simulink model "gm_soc_dvbs2_fpga"  (R2025b)
settings: Solver=VariableStepAuto  StartTime=0.0  StopTime=10.0  RelTol=1e-3
InitFcn:
  | soc_dvbs2_init;
undefined symbols (not defined in the file or in its folder): Add, coefficientsLog, coefficientsSqrt1, coefficientsSqrt2, dataBits, Deinterleaver, designMultirateFIR, noisePow, Shift, Short, soc_dvbs2_designFIRFilter, soc_dvbs2_txPacketBits, syncWord, txDataOut, txFiltCoeff, XData
libraries: simulink x304, hdlsllib x265, dspsigops x15, dsphdlfiltering2 x8, hdlmdlgenlib x6, dsphdlsigops2 x5, commseqgen3 x5, dsphdlmathfun2 x3, hwlogicconnlib x2, whdledac x2, commhdlcrc x2, whdlutilities x1
(part 31 of 36)

== system gm_soc_dvbs2_fpga/DVBS2/DVBS2 TxRx/DVB-S2 HDL Receiver/Synchronizer and PL Header Decoder/PL Header Recovery/PL Header Decoder/ML Decoder/Get Min Index/For Each Subsystem2_instance6 ==
  note: For Each
  valueIn : Inport  OutDataTypeStr=fixdt(1, 25, 15)  PortDimensions=[2]  SampleTime=2.5e-07
  idxIn : Inport  Port=2  OutDataTypeStr=fixdt(0, 6, 0)  PortDimensions=[2]  SampleTime=2.5e-07
  Delay{1..9} (9 alike) : Delay  DelayLength=double(1)  InitialCondition=0  SampleTime=2.5e-07
  Relational Operator : RelationalOperator  Operator=<  OutDataTypeStr=boolean  SampleTime=2.5e-07  InputSameDT=off
  Switch : Switch  Criteria=u2 ~= 0  Threshold="fi(0,0,1,0,\"hex\",\"0\")"  OutDataTypeStr=fixdt(1, 25, 15)  SampleTime=2.5e-07  SaturateOnIntegerOverflow=off  InputSameDT=off
  Switch1 : Switch  Criteria=u2 ~= 0  Threshold="fi(0,0,1,0,\"hex\",\"0\")"  OutDataTypeStr=fixdt(0, 6, 0)  SampleTime=2.5e-07  SaturateOnIntegerOverflow=off  InputSameDT=off
  t : Demux  Outputs=2
  t1 : Demux  Outputs=2
  ValueOut : Outport  SampleTime=2.5e-07
  idxOut : Outport  Port=2  SampleTime=2.5e-07
  wires:
  valueIn/1 -> Delay3/1
  Delay9/1 -> idxOut/1
  Delay1/1 -> t/1
  Delay3/1 -> t1/1
  idxIn/1 -> Delay1/1
  t1/1 -> Relational Operator/1, Delay4/1
  t1/2 -> Delay5/1, Relational Operator/2
  Relational Operator/1 -> Delay2/1
  Delay4/1 -> Switch/1
  t/1 -> Delay6/1
  t/2 -> Delay7/1
  Delay5/1 -> Switch/3
  Delay2/1 -> Switch/2, Switch1/2
  Delay6/1 -> Switch1/1
  Switch1/1 -> Delay9/1
  Delay7/1 -> Switch1/3
  Delay8/1 -> ValueOut/1
  Switch/1 -> Delay8/1

== system gm_soc_dvbs2_fpga/DVBS2/DVBS2 TxRx/DVB-S2 HDL Receiver/Synchronizer and PL Header Decoder/PL Header Recovery/PL Header Decoder/ML Decoder/Get Min Index/For Each Subsystem2_instance7 ==
  note: For Each
  valueIn : Inport  OutDataTypeStr=fixdt(1, 25, 15)  PortDimensions=[2]  SampleTime=2.5e-07
  idxIn : Inport  Port=2  OutDataTypeStr=fixdt(0, 6, 0)  PortDimensions=[2]  SampleTime=2.5e-07
  Delay{1..9} (9 alike) : Delay  DelayLength=double(1)  InitialCondition=0  SampleTime=2.5e-07
  Relational Operator : RelationalOperator  Operator=<  OutDataTypeStr=boolean  SampleTime=2.5e-07  InputSameDT=off
  Switch : Switch  Criteria=u2 ~= 0  Threshold="fi(0,0,1,0,\"hex\",\"0\")"  OutDataTypeStr=fixdt(1, 25, 15)  SampleTime=2.5e-07  SaturateOnIntegerOverflow=off  InputSameDT=off
  Switch1 : Switch  Criteria=u2 ~= 0  Threshold="fi(0,0,1,0,\"hex\",\"0\")"  OutDataTypeStr=fixdt(0, 6, 0)  SampleTime=2.5e-07  SaturateOnIntegerOverflow=off  InputSameDT=off
  t : Demux  Outputs=2
  t1 : Demux  Outputs=2
  ValueOut : Outport  SampleTime=2.5e-07
  idxOut : Outport  Port=2  SampleTime=2.5e-07
  wires:
  Delay8/1 -> ValueOut/1
  valueIn/1 -> Delay3/1
  idxIn/1 -> Delay1/1
  t/1 -> Delay6/1
  Switch1/1 -> Delay9/1
  t1/1 -> Delay4/1, Relational Operator/1
  Delay1/1 -> t/1
  Delay3/1 -> t1/1
  t/2 -> Delay7/1
  t1/2 -> Relational Operator/2, Delay5/1
  Relational Operator/1 -> Delay2/1
  Delay5/1 -> Switch/3
  Delay6/1 -> Switch1/1
  Delay7/1 -> Switch1/3
  Delay2/1 -> Switch/2, Switch1/2
  Delay4/1 -> Switch/1
  Switch/1 -> Delay8/1
  Delay9/1 -> idxOut/1

== system gm_soc_dvbs2_fpga/DVBS2/DVBS2 TxRx/DVB-S2 HDL Receiver/Synchronizer and PL Header Decoder/PL Header Recovery/PL Header Decoder/ML Decoder/Get Min Index/For Each Subsystem2_instance8 ==
  note: For Each
  valueIn : Inport  OutDataTypeStr=fixdt(1, 25, 15)  PortDimensions=[2]  SampleTime=2.5e-07
  idxIn : Inport  Port=2  OutDataTypeStr=fixdt(0, 6, 0)  PortDimensions=[2]  SampleTime=2.5e-07
  Delay{1..9} (9 alike) : Delay  DelayLength=double(1)  InitialCondition=0  SampleTime=2.5e-07
  Relational Operator : RelationalOperator  Operator=<  OutDataTypeStr=boolean  SampleTime=2.5e-07  InputSameDT=off
  Switch : Switch  Criteria=u2 ~= 0  Threshold="fi(0,0,1,0,\"hex\",\"0\")"  OutDataTypeStr=fixdt(1, 25, 15)  SampleTime=2.5e-07  SaturateOnIntegerOverflow=off  InputSameDT=off
  Switch1 : Switch  Criteria=u2 ~= 0  Threshold="fi(0,0,1,0,\"hex\",\"0\")"  OutDataTypeStr=fixdt(0, 6, 0)  SampleTime=2.5e-07  SaturateOnIntegerOverflow=off  InputSameDT=off
  t : Demux  Outputs=2
  t1 : Demux  Outputs=2
  ValueOut : Outport  SampleTime=2.5e-07
  idxOut : Outport  Port=2  SampleTime=2.5e-07
  wires:
  Delay8/1 -> ValueOut/1
  valueIn/1 -> Delay3/1
  idxIn/1 -> Delay1/1
  t/1 -> Delay6/1
  Switch1/1 -> Delay9/1
  t1/1 -> Delay4/1, Relational Operator/1
  Delay1/1 -> t/1
  Delay3/1 -> t1/1
  t/2 -> Delay7/1
  Delay4/1 -> Switch/1
  t1/2 -> Relational Operator/2, Delay5/1
  Relational Operator/1 -> Delay2/1
  Delay5/1 -> Switch/3
  Delay6/1 -> Switch1/1
  Delay7/1 -> Switch1/3
  Delay2/1 -> Switch/2, Switch1/2
  Switch/1 -> Delay8/1
  Delay9/1 -> idxOut/1

== system gm_soc_dvbs2_fpga/DVBS2/DVBS2 TxRx/DVB-S2 HDL Receiver/Synchronizer and PL Header Decoder/PL Header Recovery/PL Header Decoder/ML Decoder/Get Min Index/For Each Subsystem3_instance1 ==
  note: For Each
  valueIn : Inport  OutDataTypeStr=fixdt(1, 25, 15)  PortDimensions=[2]  SampleTime=2.5e-07
  idxIn : Inport  Port=2  OutDataTypeStr=fixdt(0, 6, 0)  PortDimensions=[2]  SampleTime=2.5e-07
  Delay{1..9} (9 alike) : Delay  DelayLength=double(1)  InitialCondition=0  SampleTime=2.5e-07
  Relational Operator : RelationalOperator  Operator=<  OutDataTypeStr=boolean  SampleTime=2.5e-07  InputSameDT=off
  Switch : Switch  Criteria=u2 ~= 0  Threshold="fi(0,0,1,0,\"hex\",\"0\")"  OutDataTypeStr=fixdt(1, 25, 15)  SampleTime=2.5e-07  SaturateOnIntegerOverflow=off  InputSameDT=off
  Switch1 : Switch  Criteria=u2 ~= 0  Threshold="fi(0,0,1,0,\"hex\",\"0\")"  OutDataTypeStr=fixdt(0, 6, 0)  SampleTime=2.5e-07  SaturateOnIntegerOverflow=off  InputSameDT=off
  t : Demux  Outputs=2
  t1 : Demux  Outputs=2
  ValueOut : Outport  SampleTime=2.5e-07
  idxOut : Outport  Port=2  SampleTime=2.5e-07
  wires:
  Delay4/1 -> Switch/1
  Delay8/1 -> ValueOut/1
  valueIn/1 -> Delay3/1
  Delay1/1 -> t/1
  Delay7/1 -> Switch1/3
  idxIn/1 -> Delay1/1
  Delay3/1 -> t1/1
  Switch1/1 -> Delay9/1
  t1/1 -> Relational Operator/1, Delay4/1
  Relational Operator/1 -> Delay2/1
  t1/2 -> Delay5/1, Relational Operator/2
  t/1 -> Delay6/1
  t/2 -> Delay7/1
  Delay5/1 -> Switch/3
  Delay2/1 -> Switch/2, Switch1/2
  Delay6/1 -> Switch1/1
  Switch/1 -> Delay8/1
  Delay9/1 -> idxOut/1

== system gm_soc_dvbs2_fpga/DVBS2/DVBS2 TxRx/DVB-S2 HDL Receiver/Synchronizer and PL Header Decoder/PL Header Recovery/PL Header Decoder/ML Decoder/Get Min Index/For Each Subsystem3_instance2 ==
  note: For Each
  valueIn : Inport  OutDataTypeStr=fixdt(1, 25, 15)  PortDimensions=[2]  SampleTime=2.5e-07
  idxIn : Inport  Port=2  OutDataTypeStr=fixdt(0, 6, 0)  PortDimensions=[2]  SampleTime=2.5e-07
  Delay{1..9} (9 alike) : Delay  DelayLength=double(1)  InitialCondition=0  SampleTime=2.5e-07
  Relational Operator : RelationalOperator  Operator=<  OutDataTypeStr=boolean  SampleTime=2.5e-07  InputSameDT=off
  Switch : Switch  Criteria=u2 ~= 0  Threshold="fi(0,0,1,0,\"hex\",\"0\")"  OutDataTypeStr=fixdt(1, 25, 15)  SampleTime=2.5e-07  SaturateOnIntegerOverflow=off  InputSameDT=off
  Switch1 : Switch  Criteria=u2 ~= 0  Threshold="fi(0,0,1,0,\"hex\",\"0\")"  OutDataTypeStr=fixdt(0, 6, 0)  SampleTime=2.5e-07  SaturateOnIntegerOverflow=off  InputSameDT=off
  t : Demux  Outputs=2
  t1 : Demux  Outputs=2
  ValueOut : Outport  SampleTime=2.5e-07
  idxOut : Outport  Port=2  SampleTime=2.5e-07
  wires:
  Delay8/1 -> ValueOut/1
  valueIn/1 -> Delay3/1
  Delay1/1 -> t/1
  Switch1/1 -> Delay9/1
  t1/1 -> Relational Operator/1, Delay4/1
  Delay3/1 -> t1/1
  idxIn/1 -> Delay1/1
  Relational Operator/1 -> Delay2/1
  t1/2 -> Delay5/1, Relational Operator/2
  Delay4/1 -> Switch/1
  t/1 -> Delay6/1
  t/2 -> Delay7/1
  Delay5/1 -> Switch/3
  Delay2/1 -> Switch/2, Switch1/2
  Delay6/1 -> Switch1/1
  Delay7/1 -> Switch1/3
  Switch/1 -> Delay8/1
  Delay9/1 -> idxOut/1

== system gm_soc_dvbs2_fpga/DVBS2/DVBS2 TxRx/DVB-S2 HDL Receiver/Synchronizer and PL Header Decoder/PL Header Recovery/PL Header Decoder/ML Decoder/Get Min Index/For Each Subsystem3_instance3 ==
  note: For Each
  valueIn : Inport  OutDataTypeStr=fixdt(1, 25, 15)  PortDimensions=[2]  SampleTime=2.5e-07
  idxIn : Inport  Port=2  OutDataTypeStr=fixdt(0, 6, 0)  PortDimensions=[2]  SampleTime=2.5e-07
  Delay{1..9} (9 alike) : Delay  DelayLength=double(1)  InitialCondition=0  SampleTime=2.5e-07
  Relational Operator : RelationalOperator  Operator=<  OutDataTypeStr=boolean  SampleTime=2.5e-07  InputSameDT=off
  Switch : Switch  Criteria=u2 ~= 0  Threshold="fi(0,0,1,0,\"hex\",\"0\")"  OutDataTypeStr=fixdt(1, 25, 15)  SampleTime=2.5e-07  SaturateOnIntegerOverflow=off  InputSameDT=off
  Switch1 : Switch  Criteria=u2 ~= 0  Threshold="fi(0,0,1,0,\"hex\",\"0\")"  OutDataTypeStr=fixdt(0, 6, 0)  SampleTime=2.5e-07  SaturateOnIntegerOverflow=off  InputSameDT=off
  t : Demux  Outputs=2
  t1 : Demux  Outputs=2
  ValueOut : Outport  SampleTime=2.5e-07
  idxOut : Outport  Port=2  SampleTime=2.5e-07
  wires:
  valueIn/1 -> Delay3/1
  Delay1/1 -> t/1
  Delay3/1 -> t1/1
  idxIn/1 -> Delay1/1
  t1/1 -> Relational Operator/1, Delay4/1
  t1/2 -> Delay5/1, Relational Operator/2
  Relational Operator/1 -> Delay2/1
  Delay4/1 -> Switch/1
  t/1 -> Delay6/1
  t/2 -> Delay7/1
  Delay5/1 -> Switch/3
  Delay2/1 -> Switch/2, Switch1/2
  Delay6/1 -> Switch1/1
  Switch1/1 -> Delay9/1
  Delay7/1 -> Switch1/3
  Delay8/1 -> ValueOut/1
  Switch/1 -> Delay8/1
  Delay9/1 -> idxOut/1

== system gm_soc_dvbs2_fpga/DVBS2/DVBS2 TxRx/DVB-S2 HDL Receiver/Synchronizer and PL Header Decoder/PL Header Recovery/PL Header Decoder/ML Decoder/Get Min Index/For Each Subsystem3_instance4 ==
  note: For Each
  valueIn : Inport  OutDataTypeStr=fixdt(1, 25, 15)  PortDimensions=[2]  SampleTime=2.5e-07
  idxIn : Inport  Port=2  OutDataTypeStr=fixdt(0, 6, 0)  PortDimensions=[2]  SampleTime=2.5e-07
  Delay{1..9} (9 alike) : Delay  DelayLength=double(1)  InitialCondition=0  SampleTime=2.5e-07
  Relational Operator : RelationalOperator  Operator=<  OutDataTypeStr=boolean  SampleTime=2.5e-07  InputSameDT=off
  Switch : Switch  Criteria=u2 ~= 0  Threshold="fi(0,0,1,0,\"hex\",\"0\")"  OutDataTypeStr=fixdt(1, 25, 15)  SampleTime=2.5e-07  SaturateOnIntegerOverflow=off  InputSameDT=off
  Switch1 : Switch  Criteria=u2 ~= 0  Threshold="fi(0,0,1,0,\"hex\",\"0\")"  OutDataTypeStr=fixdt(0, 6, 0)  SampleTime=2.5e-07  SaturateOnIntegerOverflow=off  InputSameDT=off
  t : Demux  Outputs=2
  t1 : Demux  Outputs=2
  ValueOut : Outport  SampleTime=2.5e-07
  idxOut : Outport  Port=2  SampleTime=2.5e-07
  wires:
  Delay8/1 -> ValueOut/1
  valueIn/1 -> Delay3/1
  Delay3/1 -> t1/1
  idxIn/1 -> Delay1/1
  t/1 -> Delay6/1
  Switch1/1 -> Delay9/1
  t1/1 -> Delay4/1, Relational Operator/1
  Delay1/1 -> t/1
  t/2 -> Delay7/1
  t1/2 -> Relational Operator/2, Delay5/1
  Relational Operator/1 -> Delay2/1
  Delay5/1 -> Switch/3
  Delay6/1 -> Switch1/1
  Delay7/1 -> Switch1/3
  Delay2/1 -> Switch/2, Switch1/2
  Delay4/1 -> Switch/1
  Switch/1 -> Delay8/1
  Delay9/1 -> idxOut/1

== system gm_soc_dvbs2_fpga/DVBS2/DVBS2 TxRx/DVB-S2 HDL Receiver/Synchronizer and PL Header Decoder/PL Header Recovery/PL Header Decoder/ML Decoder/Get Min Index/For Each Subsystem4_instance1 ==
  note: For Each
  valueIn : Inport  OutDataTypeStr=fixdt(1, 25, 15)  PortDimensions=[2]  SampleTime=2.5e-07
  idxIn : Inport  Port=2  OutDataTypeStr=fixdt(0, 6, 0)  PortDimensions=[2]  SampleTime=2.5e-07
  Delay{1..9} (9 alike) : Delay  DelayLength=double(1)  InitialCondition=0  SampleTime=2.5e-07
  Relational Operator : RelationalOperator  Operator=<  OutDataTypeStr=boolean  SampleTime=2.5e-07  InputSameDT=off
  Switch : Switch  Criteria=u2 ~= 0  Threshold="fi(0,0,1,0,\"hex\",\"0\")"  OutDataTypeStr=fixdt(1, 25, 15)  SampleTime=2.5e-07  SaturateOnIntegerOverflow=off  InputSameDT=off
  Switch1 : Switch  Criteria=u2 ~= 0  Threshold="fi(0,0,1,0,\"hex\",\"0\")"  OutDataTypeStr=fixdt(0, 6, 0)  SampleTime=2.5e-07  SaturateOnIntegerOverflow=off  InputSameDT=off
  t : Demux  Outputs=2
  t1 : Demux  Outputs=2
  ValueOut : Outport  SampleTime=2.5e-07
  idxOut : Outport  Port=2  SampleTime=2.5e-07
  wires:
  Delay4/1 -> Switch/1
  Delay8/1 -> ValueOut/1
  valueIn/1 -> Delay3/1
  Delay7/1 -> Switch1/3
  idxIn/1 -> Delay1/1
  Delay3/1 -> t1/1
  Delay1/1 -> t/1
  Switch1/1 -> Delay9/1
  t1/1 -> Relational Operator/1, Delay4/1
  Relational Operator/1 -> Delay2/1
  t1/2 -> Delay5/1, Relational Operator/2
  t/1 -> Delay6/1
  t/2 -> Delay7/1
  Delay5/1 -> Switch/3
  Delay2/1 -> Switch/2, Switch1/2
  Delay6/1 -> Switch1/1
  Switch/1 -> Delay8/1
  Delay9/1 -> idxOut/1

== system gm_soc_dvbs2_fpga/DVBS2/DVBS2 TxRx/DVB-S2 HDL Receiver/Synchronizer and PL Header Decoder/PL Header Recovery/PL Header Decoder/ML Decoder/Get Min Index/For Each Subsystem4_instance2 ==
  note: For Each
  valueIn : Inport  OutDataTypeStr=fixdt(1, 25, 15)  PortDimensions=[2]  SampleTime=2.5e-07
  idxIn : Inport  Port=2  OutDataTypeStr=fixdt(0, 6, 0)  PortDimensions=[2]  SampleTime=2.5e-07
  Delay{1..9} (9 alike) : Delay  DelayLength=double(1)  InitialCondition=0  SampleTime=2.5e-07
  Relational Operator : RelationalOperator  Operator=<  OutDataTypeStr=boolean  SampleTime=2.5e-07  InputSameDT=off
  Switch : Switch  Criteria=u2 ~= 0  Threshold="fi(0,0,1,0,\"hex\",\"0\")"  OutDataTypeStr=fixdt(1, 25, 15)  SampleTime=2.5e-07  SaturateOnIntegerOverflow=off  InputSameDT=off
  Switch1 : Switch  Criteria=u2 ~= 0  Threshold="fi(0,0,1,0,\"hex\",\"0\")"  OutDataTypeStr=fixdt(0, 6, 0)  SampleTime=2.5e-07  SaturateOnIntegerOverflow=off  InputSameDT=off
  t : Demux  Outputs=2
  t1 : Demux  Outputs=2
  ValueOut : Outport  SampleTime=2.5e-07
  idxOut : Outport  Port=2  SampleTime=2.5e-07
  wires:
  Delay8/1 -> ValueOut/1
  valueIn/1 -> Delay3/1
  Delay1/1 -> t/1
  Switch1/1 -> Delay9/1
  t1/1 -> Delay4/1, Relational Operator/1
  Delay3/1 -> t1/1
  idxIn/1 -> Delay1/1
  Relational Operator/1 -> Delay2/1
  t1/2 -> Delay5/1, Relational Operator/2
  Delay4/1 -> Switch/1
  t/1 -> Delay6/1
  t/2 -> Delay7/1
  Delay5/1 -> Switch/3
  Delay2/1 -> Switch/2, Switch1/2
  Delay6/1 -> Switch1/1
  Delay7/1 -> Switch1/3
  Switch/1 -> Delay8/1
  Delay9/1 -> idxOut/1

== system gm_soc_dvbs2_fpga/DVBS2/DVBS2 TxRx/DVB-S2 HDL Receiver/Synchronizer and PL Header Decoder/PL Header Recovery/PL Header Decoder/ML Decoder/Get Min Index/For Each Subsystem5 ==
  valueIn : Inport  OutDataTypeStr=fixdt(1, 25, 15)  PortDimensions=[2]  SampleTime=2.5e-07
  idxIn : Inport  Port=2  OutDataTypeStr=fixdt(0, 6, 0)  PortDimensions=[2]  SampleTime=2.5e-07
  Delay{1..6} (6 alike) : Delay  DelayLength=double(1)  InitialCondition=0  SampleTime=2.5e-07
  Relational Operator : RelationalOperator  Operator=<  OutDataTypeStr=boolean  SampleTime=2.5e-07  InputSameDT=off
  Switch1 : Switch  Criteria=u2 ~= 0  Threshold="fi(0,0,1,0,\"hex\",\"0\")"  OutDataTypeStr=fixdt(0, 6, 0)  SampleTime=2.5e-07  SaturateOnIntegerOverflow=off  InputSameDT=off
  t : Demux  Outputs=2
  t1 : Demux  Outputs=2
  idxOut : Outport  SampleTime=2.5e-07
  wires:
  Delay1/1 -> t1/1
  valueIn/1 -> Delay3/1
  Delay3/1 -> t/1
  t1/1 -> Delay2/1
  t/1 -> Relational Operator/1
  idxIn/1 -> Delay1/1
  Relational Operator/1 -> Delay4/1
  t/2 -> Relational Operator/2
  t1/2 -> Delay5/1
  Delay2/1 -> Switch1/1
  Delay4/1 -> Switch1/2
  Delay5/1 -> Switch1/3
  Switch1/1 -> Delay6/1
  Delay6/1 -> idxOut/1

== system gm_soc_dvbs2_fpga/DVBS2/DVBS2 TxRx/DVB-S2 HDL Receiver/Synchronizer and PL Header Decoder/PL Header Recovery/PL Header Decoder/ML Decoder/Get Min Index/For Each Subsystem_instance1 ==
  note: For Each
  valueIn : Inport  OutDataTypeStr=fixdt(1, 25, 15)  PortDimensions=[2]  SampleTime=2.5e-07
  idxIn : Inport  Port=2  OutDataTypeStr=fixdt(0, 6, 0)  PortDimensions=[2]  SampleTime=2.5e-07
  Delay{1..9} (9 alike) : Delay  DelayLength=double(1)  InitialCondition=0  SampleTime=2.5e-07
  Relational Operator : RelationalOperator  Operator=<  OutDataTypeStr=boolean  SampleTime=2.5e-07  InputSameDT=off
  Switch : Switch  Criteria=u2 ~= 0  Threshold="fi(0,0,1,0,\"hex\",\"0\")"  OutDataTypeStr=fixdt(1, 25, 15)  SampleTime=2.5e-07  SaturateOnIntegerOverflow=off  InputSameDT=off
  Switch1 : Switch  Criteria=u2 ~= 0  Threshold="fi(0,0,1,0,\"hex\",\"0\")"  OutDataTypeStr=fixdt(0, 6, 0)  SampleTime=2.5e-07  SaturateOnIntegerOverflow=off  InputSameDT=off
  t : Demux  Outputs=2
  t1 : Demux  Outputs=2
  ValueOut : Outport  SampleTime=2.5e-07
  idxOut : Outport  Port=2  SampleTime=2.5e-07
  wires:
  valueIn/1 -> Delay3/1
  Delay9/1 -> idxOut/1
  Delay1/1 -> t/1
  Switch1/1 -> Delay9/1
  t1/1 -> Relational Operator/1, Delay4/1
  Delay3/1 -> t1/1
  idxIn/1 -> Delay1/1
  Relational Operator/1 -> Delay2/1
  t1/2 -> Delay5/1, Relational Operator/2
  Delay4/1 -> Switch/1
  t/1 -> Delay6/1
  t/2 -> Delay7/1
  Delay5/1 -> Switch/3
  Delay2/1 -> Switch1/2, Switch/2
  Delay6/1 -> Switch1/1
  Delay7/1 -> Switch1/3
  Delay8/1 -> ValueOut/1
  Switch/1 -> Delay8/1

== system gm_soc_dvbs2_fpga/DVBS2/DVBS2 TxRx/DVB-S2 HDL Receiver/Synchronizer and PL Header Decoder/PL Header Recovery/PL Header Decoder/ML Decoder/Get Min Index/For Each Subsystem_instance10 ==
  note: For Each
  valueIn : Inport  OutDataTypeStr=fixdt(1, 25, 15)  PortDimensions=[2]  SampleTime=2.5e-07
  idxIn : Inport  Port=2  OutDataTypeStr=fixdt(0, 6, 0)  PortDimensions=[2]  SampleTime=2.5e-07
  Delay{1..9} (9 alike) : Delay  DelayLength=double(1)  InitialCondition=0  SampleTime=2.5e-07
  Relational Operator : RelationalOperator  Operator=<  OutDataTypeStr=boolean  SampleTime=2.5e-07  InputSameDT=off
  Switch : Switch  Criteria=u2 ~= 0  Threshold="fi(0,0,1,0,\"hex\",\"0\")"  OutDataTypeStr=fixdt(1, 25, 15)  SampleTime=2.5e-07  SaturateOnIntegerOverflow=off  InputSameDT=off
  Switch1 : Switch  Criteria=u2 ~= 0  Threshold="fi(0,0,1,0,\"hex\",\"0\")"  OutDataTypeStr=fixdt(0, 6, 0)  SampleTime=2.5e-07  SaturateOnIntegerOverflow=off  InputSameDT=off
  t : Demux  Outputs=2
  t1 : Demux  Outputs=2
  ValueOut : Outport  SampleTime=2.5e-07
  idxOut : Outport  Port=2  SampleTime=2.5e-07
  wires:
  Delay8/1 -> ValueOut/1
  valueIn/1 -> Delay3/1
  Delay1/1 -> t/1
  Switch1/1 -> Delay9/1
  t1/1 -> Relational Operator/1, Delay4/1
  Delay3/1 -> t1/1
  idxIn/1 -> Delay1/1
  Relational Operator/1 -> Delay2/1
  t1/2 -> Delay5/1, Relational Operator/2
  Delay4/1 -> Switch/1
  t/1 -> Delay6/1
  t/2 -> Delay7/1
  Delay5/1 -> Switch/3
  Delay2/1 -> Switch/2, Switch1/2
  Delay6/1 -> Switch1/1
  Delay7/1 -> Switch1/3
  Switch/1 -> Delay8/1
  Delay9/1 -> idxOut/1

== system gm_soc_dvbs2_fpga/DVBS2/DVBS2 TxRx/DVB-S2 HDL Receiver/Synchronizer and PL Header Decoder/PL Header Recovery/PL Header Decoder/ML Decoder/Get Min Index/For Each Subsystem_instance11 ==
  note: For Each
  valueIn : Inport  OutDataTypeStr=fixdt(1, 25, 15)  PortDimensions=[2]  SampleTime=2.5e-07
  idxIn : Inport  Port=2  OutDataTypeStr=fixdt(0, 6, 0)  PortDimensions=[2]  SampleTime=2.5e-07
  Delay{1..9} (9 alike) : Delay  DelayLength=double(1)  InitialCondition=0  SampleTime=2.5e-07
  Relational Operator : RelationalOperator  Operator=<  OutDataTypeStr=boolean  SampleTime=2.5e-07  InputSameDT=off
  Switch : Switch  Criteria=u2 ~= 0  Threshold="fi(0,0,1,0,\"hex\",\"0\")"  OutDataTypeStr=fixdt(1, 25, 15)  SampleTime=2.5e-07  SaturateOnIntegerOverflow=off  InputSameDT=off
  Switch1 : Switch  Criteria=u2 ~= 0  Threshold="fi(0,0,1,0,\"hex\",\"0\")"  OutDataTypeStr=fixdt(0, 6, 0)  SampleTime=2.5e-07  SaturateOnIntegerOverflow=off  InputSameDT=off
  t : Demux  Outputs=2
  t1 : Demux  Outputs=2
  ValueOut : Outport  SampleTime=2.5e-07
  idxOut : Outport  Port=2  SampleTime=2.5e-07
  wires:
  Delay8/1 -> ValueOut/1
  valueIn/1 -> Delay3/1
  Delay9/1 -> idxOut/1
  Delay1/1 -> t/1
  Delay3/1 -> t1/1
  idxIn/1 -> Delay1/1
  t/1 -> Delay6/1
  Switch1/1 -> Delay9/1
  t1/1 -> Delay4/1, Relational Operator/1
  t/2 -> Delay7/1
  t1/2 -> Relational Operator/2, Delay5/1
  Relational Operator/1 -> Delay2/1
  Delay5/1 -> Switch/3
  Delay6/1 -> Switch1/1
  Delay7/1 -> Switch1/3
  Delay2/1 -> Switch/2, Switch1/2
  Delay4/1 -> Switch/1
  Switch/1 -> Delay8/1

== system gm_soc_dvbs2_fpga/DVBS2/DVBS2 TxRx/DVB-S2 HDL Receiver/Synchronizer and PL Header Decoder/PL Header Recovery/PL Header Decoder/ML Decoder/Get Min Index/For Each Subsystem_instance12 ==
  note: For Each
  valueIn : Inport  OutDataTypeStr=fixdt(1, 25, 15)  PortDimensions=[2]  SampleTime=2.5e-07
  idxIn : Inport  Port=2  OutDataTypeStr=fixdt(0, 6, 0)  PortDimensions=[2]  SampleTime=2.5e-07
  Delay{1..9} (9 alike) : Delay  DelayLength=double(1)  InitialCondition=0  SampleTime=2.5e-07
  Relational Operator : RelationalOperator  Operator=<  OutDataTypeStr=boolean  SampleTime=2.5e-07  InputSameDT=off
  Switch : Switch  Criteria=u2 ~= 0  Threshold="fi(0,0,1,0,\"hex\",\"0\")"  OutDataTypeStr=fixdt(1, 25, 15)  SampleTime=2.5e-07  SaturateOnIntegerOverflow=off  InputSameDT=off
  Switch1 : Switch  Criteria=u2 ~= 0  Threshold="fi(0,0,1,0,\"hex\",\"0\")"  OutDataTypeStr=fixdt(0, 6, 0)  SampleTime=2.5e-07  SaturateOnIntegerOverflow=off  InputSameDT=off
  t : Demux  Outputs=2
  t1 : Demux  Outputs=2
  ValueOut : Outport  SampleTime=2.5e-07
  idxOut : Outport  Port=2  SampleTime=2.5e-07
  wires:
  Delay8/1 -> ValueOut/1
  valueIn/1 -> Delay3/1
  Delay1/1 -> t/1
  Switch1/1 -> Delay9/1
  t1/1 -> Relational Operator/1, Delay4/1
  Delay3/1 -> t1/1
  idxIn/1 -> Delay1/1
  Relational Operator/1 -> Delay2/1
  t1/2 -> Delay5/1, Relational Operator/2
  Delay4/1 -> Switch/1
  t/1 -> Delay6/1
  t/2 -> Delay7/1
  Delay5/1 -> Switch/3
  Delay2/1 -> Switch/2, Switch1/2
  Delay6/1 -> Switch1/1
  Delay7/1 -> Switch1/3
  Switch/1 -> Delay8/1
  Delay9/1 -> idxOut/1

== system gm_soc_dvbs2_fpga/DVBS2/DVBS2 TxRx/DVB-S2 HDL Receiver/Synchronizer and PL Header Decoder/PL Header Recovery/PL Header Decoder/ML Decoder/Get Min Index/For Each Subsystem_instance13 ==
  note: For Each
  valueIn : Inport  OutDataTypeStr=fixdt(1, 25, 15)  PortDimensions=[2]  SampleTime=2.5e-07
  idxIn : Inport  Port=2  OutDataTypeStr=fixdt(0, 6, 0)  PortDimensions=[2]  SampleTime=2.5e-07
  Delay{1..9} (9 alike) : Delay  DelayLength=double(1)  InitialCondition=0  SampleTime=2.5e-07
  Relational Operator : RelationalOperator  Operator=<  OutDataTypeStr=boolean  SampleTime=2.5e-07  InputSameDT=off
  Switch : Switch  Criteria=u2 ~= 0  Threshold="fi(0,0,1,0,\"hex\",\"0\")"  OutDataTypeStr=fixdt(1, 25, 15)  SampleTime=2.5e-07  SaturateOnIntegerOverflow=off  InputSameDT=off
  Switch1 : Switch  Criteria=u2 ~= 0  Threshold="fi(0,0,1,0,\"hex\",\"0\")"  OutDataTypeStr=fixdt(0, 6, 0)  SampleTime=2.5e-07  SaturateOnIntegerOverflow=off  InputSameDT=off
  t : Demux  Outputs=2
  t1 : Demux  Outputs=2
  ValueOut : Outport  SampleTime=2.5e-07
  idxOut : Outport  Port=2  SampleTime=2.5e-07
  wires:
  valueIn/1 -> Delay3/1
  idxIn/1 -> Delay1/1
  t/1 -> Delay6/1
  Delay1/1 -> t/1
  Delay3/1 -> t1/1
  t1/1 -> Delay4/1, Relational Operator/1
  t/2 -> Delay7/1
  t1/2 -> Relational Operator/2, Delay5/1
  Relational Operator/1 -> Delay2/1
  Delay5/1 -> Switch/3
  Delay6/1 -> Switch1/1
  Switch1/1 -> Delay9/1
  Delay7/1 -> Switch1/3
  Delay2/1 -> Switch/2, Switch1/2
  Delay4/1 -> Switch/1
  Delay8/1 -> ValueOut/1
  Switch/1 -> Delay8/1
  Delay9/1 -> idxOut/1

== system gm_soc_dvbs2_fpga/DVBS2/DVBS2 TxRx/DVB-S2 HDL Receiver/Synchronizer and PL Header Decoder/PL Header Recovery/PL Header Decoder/ML Decoder/Get Min Index/For Each Subsystem_instance14 ==
  note: For Each
  valueIn : Inport  OutDataTypeStr=fixdt(1, 25, 15)  PortDimensions=[2]  SampleTime=2.5e-07
  idxIn : Inport  Port=2  OutDataTypeStr=fixdt(0, 6, 0)  PortDimensions=[2]  SampleTime=2.5e-07
  Delay{1..9} (9 alike) : Delay  DelayLength=double(1)  InitialCondition=0  SampleTime=2.5e-07
  Relational Operator : RelationalOperator  Operator=<  OutDataTypeStr=boolean  SampleTime=2.5e-07  InputSameDT=off
  Switch : Switch  Criteria=u2 ~= 0  Threshold="fi(0,0,1,0,\"hex\",\"0\")"  OutDataTypeStr=fixdt(1, 25, 15)  SampleTime=2.5e-07  SaturateOnIntegerOverflow=off  InputSameDT=off
  Switch1 : Switch  Criteria=u2 ~= 0  Threshold="fi(0,0,1,0,\"hex\",\"0\")"  OutDataTypeStr=fixdt(0, 6, 0)  SampleTime=2.5e-07  SaturateOnIntegerOverflow=off  InputSameDT=off
  t : Demux  Outputs=2
  t1 : Demux  Outputs=2
  ValueOut : Outport  SampleTime=2.5e-07
  idxOut : Outport  Port=2  SampleTime=2.5e-07
  wires:
  Delay8/1 -> ValueOut/1
  valueIn/1 -> Delay3/1
  Delay3/1 -> t1/1
  idxIn/1 -> Delay1/1
  t/1 -> Delay6/1
  Switch1/1 -> Delay9/1
  t1/1 -> Delay4/1, Relational Operator/1
  Delay1/1 -> t/1
  t/2 -> Delay7/1
  t1/2 -> Relational Operator/2, Delay5/1
  Relational Operator/1 -> Delay2/1
  Delay5/1 -> Switch/3
  Delay6/1 -> Switch1/1
  Delay7/1 -> Switch1/3
  Delay2/1 -> Switch/2, Switch1/2
  Delay4/1 -> Switch/1
  Switch/1 -> Delay8/1
  Delay9/1 -> idxOut/1

== system gm_soc_dvbs2_fpga/DVBS2/DVBS2 TxRx/DVB-S2 HDL Receiver/Synchronizer and PL Header Decoder/PL Header Recovery/PL Header Decoder/ML Decoder/Get Min Index/For Each Subsystem_instance15 ==
  note: For Each
  valueIn : Inport  OutDataTypeStr=fixdt(1, 25, 15)  PortDimensions=[2]  SampleTime=2.5e-07
  idxIn : Inport  Port=2  OutDataTypeStr=fixdt(0, 6, 0)  PortDimensions=[2]  SampleTime=2.5e-07
  Delay{1..9} (9 alike) : Delay  DelayLength=double(1)  InitialCondition=0  SampleTime=2.5e-07
  Relational Operator : RelationalOperator  Operator=<  OutDataTypeStr=boolean  SampleTime=2.5e-07  InputSameDT=off
  Switch : Switch  Criteria=u2 ~= 0  Threshold="fi(0,0,1,0,\"hex\",\"0\")"  OutDataTypeStr=fixdt(1, 25, 15)  SampleTime=2.5e-07  SaturateOnIntegerOverflow=off  InputSameDT=off
  Switch1 : Switch  Criteria=u2 ~= 0  Threshold="fi(0,0,1,0,\"hex\",\"0\")"  OutDataTypeStr=fixdt(0, 6, 0)  SampleTime=2.5e-07  SaturateOnIntegerOverflow=off  InputSameDT=off
  t : Demux  Outputs=2
  t1 : Demux  Outputs=2
  ValueOut : Outport  SampleTime=2.5e-07
  idxOut : Outport  Port=2  SampleTime=2.5e-07
  wires:
  Delay8/1 -> ValueOut/1
  valueIn/1 -> Delay3/1
  Delay1/1 -> t/1
  Switch1/1 -> Delay9/1
  t1/1 -> Relational Operator/1, Delay4/1
  Delay3/1 -> t1/1
  idxIn/1 -> Delay1/1
  Relational Operator/1 -> Delay2/1
  t1/2 -> Delay5/1, Relational Operator/2
  Delay4/1 -> Switch/1
  t/1 -> Delay6/1
  t/2 -> Delay7/1
  Delay5/1 -> Switch/3
  Delay2/1 -> Switch1/2, Switch/2
  Delay6/1 -> Switch1/1
  Delay7/1 -> Switch1/3
  Switch/1 -> Delay8/1
  Delay9/1 -> idxOut/1

== system gm_soc_dvbs2_fpga/DVBS2/DVBS2 TxRx/DVB-S2 HDL Receiver/Synchronizer and PL Header Decoder/PL Header Recovery/PL Header Decoder/ML Decoder/Get Min Index/For Each Subsystem_instance16 ==
  note: For Each
  valueIn : Inport  OutDataTypeStr=fixdt(1, 25, 15)  PortDimensions=[2]  SampleTime=2.5e-07
  idxIn : Inport  Port=2  OutDataTypeStr=fixdt(0, 6, 0)  PortDimensions=[2]  SampleTime=2.5e-07
  Delay{1..9} (9 alike) : Delay  DelayLength=double(1)  InitialCondition=0  SampleTime=2.5e-07
  Relational Operator : RelationalOperator  Operator=<  OutDataTypeStr=boolean  SampleTime=2.5e-07  InputSameDT=off
  Switch : Switch  Criteria=u2 ~= 0  Threshold="fi(0,0,1,0,\"hex\",\"0\")"  OutDataTypeStr=fixdt(1, 25, 15)  SampleTime=2.5e-07  SaturateOnIntegerOverflow=off  InputSameDT=off
  Switch1 : Switch  Criteria=u2 ~= 0  Threshold="fi(0,0,1,0,\"hex\",\"0\")"  OutDataTypeStr=fixdt(0, 6, 0)  SampleTime=2.5e-07  SaturateOnIntegerOverflow=off  InputSameDT=off
  t : Demux  Outputs=2
  t1 : Demux  Outputs=2
  ValueOut : Outport  SampleTime=2.5e-07
  idxOut : Outport  Port=2  SampleTime=2.5e-07
  wires:
  valueIn/1 -> Delay3/1
  Delay9/1 -> idxOut/1
  Delay1/1 -> t/1
  Delay3/1 -> t1/1
  idxIn/1 -> Delay1/1
  t1/1 -> Relational Operator/1, Delay4/1
  Relational Operator/1 -> Delay2/1
  t1/2 -> Delay5/1, Relational Operator/2
  Delay4/1 -> Switch/1
  t/1 -> Delay6/1
  t/2 -> Delay7/1
  Delay5/1 -> Switch/3
  Delay2/1 -> Switch/2, Switch1/2
  Delay6/1 -> Switch1/1
  Switch1/1 -> Delay9/1
  Delay7/1 -> Switch1/3
  Delay8/1 -> ValueOut/1
  Switch/1 -> Delay8/1

== system gm_soc_dvbs2_fpga/DVBS2/DVBS2 TxRx/DVB-S2 HDL Receiver/Synchronizer and PL Header Decoder/PL Header Recovery/PL Header Decoder/ML Decoder/Get Min Index/For Each Subsystem_instance17 ==
  note: For Each
  valueIn : Inport  OutDataTypeStr=fixdt(1, 25, 15)  PortDimensions=[2]  SampleTime=2.5e-07
  idxIn : Inport  Port=2  OutDataTypeStr=fixdt(0, 6, 0)  PortDimensions=[2]  SampleTime=2.5e-07
  Delay{1..9} (9 alike) : Delay  DelayLength=double(1)  InitialCondition=0  SampleTime=2.5e-07
  Relational Operator : RelationalOperator  Operator=<  OutDataTypeStr=boolean  SampleTime=2.5e-07  InputSameDT=off
  Switch : Switch  Criteria=u2 ~= 0  Threshold="fi(0,0,1,0,\"hex\",\"0\")"  OutDataTypeStr=fixdt(1, 25, 15)  SampleTime=2.5e-07  SaturateOnIntegerOverflow=off  InputSameDT=off
  Switch1 : Switch  Criteria=u2 ~= 0  Threshold="fi(0,0,1,0,\"hex\",\"0\")"  OutDataTypeStr=fixdt(0, 6, 0)  SampleTime=2.5e-07  SaturateOnIntegerOverflow=off  InputSameDT=off
  t : Demux  Outputs=2
  t1 : Demux  Outputs=2
  ValueOut : Outport  SampleTime=2.5e-07
  idxOut : Outport  Port=2  SampleTime=2.5e-07
  wires:
  Delay8/1 -> ValueOut/1
  valueIn/1 -> Delay3/1
  Delay1/1 -> t/1
  Switch1/1 -> Delay9/1
  t1/1 -> Relational Operator/1, Delay4/1
  Delay3/1 -> t1/1
  idxIn/1 -> Delay1/1
  Relational Operator/1 -> Delay2/1
  t1/2 -> Delay5/1, Relational Operator/2
  Delay4/1 -> Switch/1
  t/1 -> Delay6/1
  t/2 -> Delay7/1
  Delay5/1 -> Switch/3
  Delay2/1 -> Switch/2, Switch1/2
  Delay6/1 -> Switch1/1
  Delay7/1 -> Switch1/3
  Switch/1 -> Delay8/1
  Delay9/1 -> idxOut/1

== system gm_soc_dvbs2_fpga/DVBS2/DVBS2 TxRx/DVB-S2 HDL Receiver/Synchronizer and PL Header Decoder/PL Header Recovery/PL Header Decoder/ML Decoder/Get Min Index/For Each Subsystem_instance18 ==
  note: For Each
  valueIn : Inport  OutDataTypeStr=fixdt(1, 25, 15)  PortDimensions=[2]  SampleTime=2.5e-07
  idxIn : Inport  Port=2  OutDataTypeStr=fixdt(0, 6, 0)  PortDimensions=[2]  SampleTime=2.5e-07
  Delay{1..9} (9 alike) : Delay  DelayLength=double(1)  InitialCondition=0  SampleTime=2.5e-07
  Relational Operator : RelationalOperator  Operator=<  OutDataTypeStr=boolean  SampleTime=2.5e-07  InputSameDT=off
  Switch : Switch  Criteria=u2 ~= 0  Threshold="fi(0,0,1,0,\"hex\",\"0\")"  OutDataTypeStr=fixdt(1, 25, 15)  SampleTime=2.5e-07  SaturateOnIntegerOverflow=off  InputSameDT=off
  Switch1 : Switch  Criteria=u2 ~= 0  Threshold="fi(0,0,1,0,\"hex\",\"0\")"  OutDataTypeStr=fixdt(0, 6, 0)  SampleTime=2.5e-07  SaturateOnIntegerOverflow=off  InputSameDT=off
  t : Demux  Outputs=2
  t1 : Demux  Outputs=2
  ValueOut : Outport  SampleTime=2.5e-07
  idxOut : Outport  Port=2  SampleTime=2.5e-07
  wires:
  Delay8/1 -> ValueOut/1
  valueIn/1 -> Delay3/1
  Delay1/1 -> t/1
  Switch1/1 -> Delay9/1
  t1/1 -> Relational Operator/1, Delay4/1
  Delay3/1 -> t1/1
  idxIn/1 -> Delay1/1
  Relational Operator/1 -> Delay2/1
  t1/2 -> Delay5/1, Relational Operator/2
  Delay4/1 -> Switch/1
  t/1 -> Delay6/1
  t/2 -> Delay7/1
  Delay5/1 -> Switch/3
  Delay2/1 -> Switch/2, Switch1/2
  Delay6/1 -> Switch1/1
  Delay7/1 -> Switch1/3
  Switch/1 -> Delay8/1
  Delay9/1 -> idxOut/1

== system gm_soc_dvbs2_fpga/DVBS2/DVBS2 TxRx/DVB-S2 HDL Receiver/Synchronizer and PL Header Decoder/PL Header Recovery/PL Header Decoder/ML Decoder/Get Min Index/For Each Subsystem_instance19 ==
  note: For Each
  valueIn : Inport  OutDataTypeStr=fixdt(1, 25, 15)  PortDimensions=[2]  SampleTime=2.5e-07
  idxIn : Inport  Port=2  OutDataTypeStr=fixdt(0, 6, 0)  PortDimensions=[2]  SampleTime=2.5e-07
  Delay{1..9} (9 alike) : Delay  DelayLength=double(1)  InitialCondition=0  SampleTime=2.5e-07
  Relational Operator : RelationalOperator  Operator=<  OutDataTypeStr=boolean  SampleTime=2.5e-07  InputSameDT=off
  Switch : Switch  Criteria=u2 ~= 0  Threshold="fi(0,0,1,0,\"hex\",\"0\")"  OutDataTypeStr=fixdt(1, 25, 15)  SampleTime=2.5e-07  SaturateOnIntegerOverflow=off  InputSameDT=off
  Switch1 : Switch  Criteria=u2 ~= 0  Threshold="fi(0,0,1,0,\"hex\",\"0\")"  OutDataTypeStr=fixdt(0, 6, 0)  SampleTime=2.5e-07  SaturateOnIntegerOverflow=off  InputSameDT=off
  t : Demux  Outputs=2
  t1 : Demux  Outputs=2
  ValueOut : Outport  SampleTime=2.5e-07
  idxOut : Outport  Port=2  SampleTime=2.5e-07
  wires:
  valueIn/1 -> Delay3/1
  idxIn/1 -> Delay1/1
  Delay9/1 -> idxOut/1
  Delay1/1 -> t/1
  Delay3/1 -> t1/1
  t/1 -> Delay6/1
  t1/1 -> Delay4/1, Relational Operator/1
  t/2 -> Delay7/1
  t1/2 -> Relational Operator/2, Delay5/1
  Relational Operator/1 -> Delay2/1
  Delay5/1 -> Switch/3
  Delay6/1 -> Switch1/1
  Switch1/1 -> Delay9/1
  Delay7/1 -> Switch1/3
  Delay2/1 -> Switch/2, Switch1/2
  Delay4/1 -> Switch/1
  Switch/1 -> Delay8/1
  Delay8/1 -> ValueOut/1

== system gm_soc_dvbs2_fpga/DVBS2/DVBS2 TxRx/DVB-S2 HDL Receiver/Synchronizer and PL Header Decoder/PL Header Recovery/PL Header Decoder/ML Decoder/Get Min Index/For Each Subsystem_instance2 ==
  note: For Each
  valueIn : Inport  OutDataTypeStr=fixdt(1, 25, 15)  PortDimensions=[2]  SampleTime=2.5e-07
  idxIn : Inport  Port=2  OutDataTypeStr=fixdt(0, 6, 0)  PortDimensions=[2]  SampleTime=2.5e-07
  Delay{1..9} (9 alike) : Delay  DelayLength=double(1)  InitialCondition=0  SampleTime=2.5e-07
  Relational Operator : RelationalOperator  Operator=<  OutDataTypeStr=boolean  SampleTime=2.5e-07  InputSameDT=off
  Switch : Switch  Criteria=u2 ~= 0  Threshold="fi(0,0,1,0,\"hex\",\"0\")"  OutDataTypeStr=fixdt(1, 25, 15)  SampleTime=2.5e-07  SaturateOnIntegerOverflow=off  InputSameDT=off
  Switch1 : Switch  Criteria=u2 ~= 0  Threshold="fi(0,0,1,0,\"hex\",\"0\")"  OutDataTypeStr=fixdt(0, 6, 0)  SampleTime=2.5e-07  SaturateOnIntegerOverflow=off  InputSameDT=off
  t : Demux  Outputs=2
  t1 : Demux  Outputs=2
  ValueOut : Outport  SampleTime=2.5e-07
  idxOut : Outport  Port=2  SampleTime=2.5e-07
  wires:
  valueIn/1 -> Delay3/1
  Delay9/1 -> idxOut/1
  Delay1/1 -> t/1
  Delay3/1 -> t1/1
  idxIn/1 -> Delay1/1
  t1/1 -> Relational Operator/1, Delay4/1
  t1/2 -> Delay5/1, Relational Operator/2
  Relational Operator/1 -> Delay2/1
  Delay4/1 -> Switch/1
  t/1 -> Delay6/1
  t/2 -> Delay7/1
  Delay5/1 -> Switch/3
  Delay2/1 -> Switch/2, Switch1/2
  Delay6/1 -> Switch1/1
  Switch1/1 -> Delay9/1
  Delay7/1 -> Switch1/3
  Delay8/1 -> ValueOut/1
  Switch/1 -> Delay8/1

== system gm_soc_dvbs2_fpga/DVBS2/DVBS2 TxRx/DVB-S2 HDL Receiver/Synchronizer and PL Header Decoder/PL Header Recovery/PL Header Decoder/ML Decoder/Get Min Index/For Each Subsystem_instance20 ==
  note: For Each
  valueIn : Inport  OutDataTypeStr=fixdt(1, 25, 15)  PortDimensions=[2]  SampleTime=2.5e-07
  idxIn : Inport  Port=2  OutDataTypeStr=fixdt(0, 6, 0)  PortDimensions=[2]  SampleTime=2.5e-07
  Delay{1..9} (9 alike) : Delay  DelayLength=double(1)  InitialCondition=0  SampleTime=2.5e-07
  Relational Operator : RelationalOperator  Operator=<  OutDataTypeStr=boolean  SampleTime=2.5e-07  InputSameDT=off
  Switch : Switch  Criteria=u2 ~= 0  Threshold="fi(0,0,1,0,\"hex\",\"0\")"  OutDataTypeStr=fixdt(1, 25, 15)  SampleTime=2.5e-07  SaturateOnIntegerOverflow=off  InputSameDT=off
  Switch1 : Switch  Criteria=u2 ~= 0  Threshold="fi(0,0,1,0,\"hex\",\"0\")"  OutDataTypeStr=fixdt(0, 6, 0)  SampleTime=2.5e-07  SaturateOnIntegerOverflow=off  InputSameDT=off
  t : Demux  Outputs=2
  t1 : Demux  Outputs=2
  ValueOut : Outport  SampleTime=2.5e-07
  idxOut : Outport  Port=2  SampleTime=2.5e-07
  wires:
  Delay8/1 -> ValueOut/1
  valueIn/1 -> Delay3/1
  Delay1/1 -> t/1
  Switch1/1 -> Delay9/1
  t1/1 -> Relational Operator/1, Delay4/1
  Delay3/1 -> t1/1
  idxIn/1 -> Delay1/1
  Relational Operator/1 -> Delay2/1
  t1/2 -> Delay5/1, Relational Operator/2
  Delay4/1 -> Switch/1
  t/1 -> Delay6/1
  t/2 -> Delay7/1
  Delay5/1 -> Switch/3
  Delay2/1 -> Switch/2, Switch1/2
  Delay6/1 -> Switch1/1
  Delay7/1 -> Switch1/3
  Switch/1 -> Delay8/1
  Delay9/1 -> idxOut/1

== system gm_soc_dvbs2_fpga/DVBS2/DVBS2 TxRx/DVB-S2 HDL Receiver/Synchronizer and PL Header Decoder/PL Header Recovery/PL Header Decoder/ML Decoder/Get Min Index/For Each Subsystem_instance21 ==
  note: For Each
  valueIn : Inport  OutDataTypeStr=fixdt(1, 25, 15)  PortDimensions=[2]  SampleTime=2.5e-07
  idxIn : Inport  Port=2  OutDataTypeStr=fixdt(0, 6, 0)  PortDimensions=[2]  SampleTime=2.5e-07
  Delay{1..9} (9 alike) : Delay  DelayLength=double(1)  InitialCondition=0  SampleTime=2.5e-07
  Relational Operator : RelationalOperator  Operator=<  OutDataTypeStr=boolean  SampleTime=2.5e-07  InputSameDT=off
  Switch : Switch  Criteria=u2 ~= 0  Threshold="fi(0,0,1,0,\"hex\",\"0\")"  OutDataTypeStr=fixdt(1, 25, 15)  SampleTime=2.5e-07  SaturateOnIntegerOverflow=off  InputSameDT=off
  Switch1 : Switch  Criteria=u2 ~= 0  Threshold="fi(0,0,1,0,\"hex\",\"0\")"  OutDataTypeStr=fixdt(0, 6, 0)  SampleTime=2.5e-07  SaturateOnIntegerOverflow=off  InputSameDT=off
  t : Demux  Outputs=2
  t1 : Demux  Outputs=2
  ValueOut : Outport  SampleTime=2.5e-07
  idxOut : Outport  Port=2  SampleTime=2.5e-07
  wires:
  Delay8/1 -> ValueOut/1
  valueIn/1 -> Delay3/1
  idxIn/1 -> Delay1/1
  t/1 -> Delay6/1
  Switch1/1 -> Delay9/1
  t1/1 -> Delay4/1, Relational Operator/1
  Delay1/1 -> t/1
  Delay3/1 -> t1/1
  t/2 -> Delay7/1
  Delay4/1 -> Switch/1
  t1/2 -> Relational Operator/2, Delay5/1
  Relational Operator/1 -> Delay2/1
  Delay5/1 -> Switch/3
  Delay6/1 -> Switch1/1
  Delay7/1 -> Switch1/3
  Delay2/1 -> Switch/2, Switch1/2
  Switch/1 -> Delay8/1
  Delay9/1 -> idxOut/1

== system gm_soc_dvbs2_fpga/DVBS2/DVBS2 TxRx/DVB-S2 HDL Receiver/Synchronizer and PL Header Decoder/PL Header Recovery/PL Header Decoder/ML Decoder/Get Min Index/For Each Subsystem_instance22 ==
  note: For Each
  valueIn : Inport  OutDataTypeStr=fixdt(1, 25, 15)  PortDimensions=[2]  SampleTime=2.5e-07
  idxIn : Inport  Port=2  OutDataTypeStr=fixdt(0, 6, 0)  PortDimensions=[2]  SampleTime=2.5e-07
  Delay{1..9} (9 alike) : Delay  DelayLength=double(1)  InitialCondition=0  SampleTime=2.5e-07
  Relational Operator : RelationalOperator  Operator=<  OutDataTypeStr=boolean  SampleTime=2.5e-07  InputSameDT=off
  Switch : Switch  Criteria=u2 ~= 0  Threshold="fi(0,0,1,0,\"hex\",\"0\")"  OutDataTypeStr=fixdt(1, 25, 15)  SampleTime=2.5e-07  SaturateOnIntegerOverflow=off  InputSameDT=off
  Switch1 : Switch  Criteria=u2 ~= 0  Threshold="fi(0,0,1,0,\"hex\",\"0\")"  OutDataTypeStr=fixdt(0, 6, 0)  SampleTime=2.5e-07  SaturateOnIntegerOverflow=off  InputSameDT=off
  t : Demux  Outputs=2
  t1 : Demux  Outputs=2
  ValueOut : Outport  SampleTime=2.5e-07
  idxOut : Outport  Port=2  SampleTime=2.5e-07
  wires:
  valueIn/1 -> Delay3/1
  Delay9/1 -> idxOut/1
  Delay1/1 -> t/1
  idxIn/1 -> Delay1/1
  Delay3/1 -> t1/1
  Switch1/1 -> Delay9/1
  t1/1 -> Relational Operator/1, Delay4/1
  Relational Operator/1 -> Delay2/1
  t1/2 -> Delay5/1, Relational Operator/2
  Delay4/1 -> Switch/1
  t/1 -> Delay6/1
  t/2 -> Delay7/1
  Delay5/1 -> Switch/3
  Delay2/1 -> Switch/2, Switch1/2
  Delay6/1 -> Switch1/1
  Delay7/1 -> Switch1/3
  Switch/1 -> Delay8/1
  Delay8/1 -> ValueOut/1

== system gm_soc_dvbs2_fpga/DVBS2/DVBS2 TxRx/DVB-S2 HDL Receiver/Synchronizer and PL Header Decoder/PL Header Recovery/PL Header Decoder/ML Decoder/Get Min Index/For Each Subsystem_instance23 ==
  note: For Each
  valueIn : Inport  OutDataTypeStr=fixdt(1, 25, 15)  PortDimensions=[2]  SampleTime=2.5e-07
  idxIn : Inport  Port=2  OutDataTypeStr=fixdt(0, 6, 0)  PortDimensions=[2]  SampleTime=2.5e-07
  Delay{1..9} (9 alike) : Delay  DelayLength=double(1)  InitialCondition=0  SampleTime=2.5e-07
  Relational Operator : RelationalOperator  Operator=<  OutDataTypeStr=boolean  SampleTime=2.5e-07  InputSameDT=off
  Switch : Switch  Criteria=u2 ~= 0  Threshold="fi(0,0,1,0,\"hex\",\"0\")"  OutDataTypeStr=fixdt(1, 25, 15)  SampleTime=2.5e-07  SaturateOnIntegerOverflow=off  InputSameDT=off
  Switch1 : Switch  Criteria=u2 ~= 0  Threshold="fi(0,0,1,0,\"hex\",\"0\")"  OutDataTypeStr=fixdt(0, 6, 0)  SampleTime=2.5e-07  SaturateOnIntegerOverflow=off  InputSameDT=off
  t : Demux  Outputs=2
  t1 : Demux  Outputs=2
  ValueOut : Outport  SampleTime=2.5e-07
  idxOut : Outport  Port=2  SampleTime=2.5e-07
  wires:
  Delay8/1 -> ValueOut/1
  valueIn/1 -> Delay3/1
  idxIn/1 -> Delay1/1
  t/1 -> Delay6/1
  Switch1/1 -> Delay9/1
  t1/1 -> Delay4/1, Relational Operator/1
  Delay1/1 -> t/1
  Delay3/1 -> t1/1
  t/2 -> Delay7/1
  Delay4/1 -> Switch/1
  t1/2 -> Relational Operator/2, Delay5/1
  Relational Operator/1 -> Delay2/1
  Delay5/1 -> Switch/3
  Delay6/1 -> Switch1/1
  Delay7/1 -> Switch1/3
  Delay2/1 -> Switch/2, Switch1/2
  Switch/1 -> Delay8/1
  Delay9/1 -> idxOut/1

== system gm_soc_dvbs2_fpga/DVBS2/DVBS2 TxRx/DVB-S2 HDL Receiver/Synchronizer and PL Header Decoder/PL Header Recovery/PL Header Decoder/ML Decoder/Get Min Index/For Each Subsystem_instance24 ==
  note: For Each
  valueIn : Inport  OutDataTypeStr=fixdt(1, 25, 15)  PortDimensions=[2]  SampleTime=2.5e-07
  idxIn : Inport  Port=2  OutDataTypeStr=fixdt(0, 6, 0)  PortDimensions=[2]  SampleTime=2.5e-07
  Delay{1..9} (9 alike) : Delay  DelayLength=double(1)  InitialCondition=0  SampleTime=2.5e-07
  Relational Operator : RelationalOperator  Operator=<  OutDataTypeStr=boolean  SampleTime=2.5e-07  InputSameDT=off
  Switch : Switch  Criteria=u2 ~= 0  Threshold="fi(0,0,1,0,\"hex\",\"0\")"  OutDataTypeStr=fixdt(1, 25, 15)  SampleTime=2.5e-07  SaturateOnIntegerOverflow=off  InputSameDT=off
  Switch1 : Switch  Criteria=u2 ~= 0  Threshold="fi(0,0,1,0,\"hex\",\"0\")"  OutDataTypeStr=fixdt(0, 6, 0)  SampleTime=2.5e-07  SaturateOnIntegerOverflow=off  InputSameDT=off
  t : Demux  Outputs=2
  t1 : Demux  Outputs=2
  ValueOut : Outport  SampleTime=2.5e-07
  idxOut : Outport  Port=2  SampleTime=2.5e-07
  wires:
  Delay8/1 -> ValueOut/1
  valueIn/1 -> Delay3/1
  Delay1/1 -> t/1
  Delay3/1 -> t1/1
  idxIn/1 -> Delay1/1
  t1/1 -> Relational Operator/1, Delay4/1
  t1/2 -> Delay5/1, Relational Operator/2
  Relational Operator/1 -> Delay2/1
  Delay4/1 -> Switch/1
  t/1 -> Delay6/1
  t/2 -> Delay7/1
  Delay5/1 -> Switch/3
  Delay2/1 -> Switch1/2, Switch/2
  Delay6/1 -> Switch1/1
  Switch1/1 -> Delay9/1
  Delay7/1 -> Switch1/3
  Switch/1 -> Delay8/1
  Delay9/1 -> idxOut/1

== system gm_soc_dvbs2_fpga/DVBS2/DVBS2 TxRx/DVB-S2 HDL Receiver/Synchronizer and PL Header Decoder/PL Header Recovery/PL Header Decoder/ML Decoder/Get Min Index/For Each Subsystem_instance25 ==
  note: For Each
  valueIn : Inport  OutDataTypeStr=fixdt(1, 25, 15)  PortDimensions=[2]  SampleTime=2.5e-07
  idxIn : Inport  Port=2  OutDataTypeStr=fixdt(0, 6, 0)  PortDimensions=[2]  SampleTime=2.5e-07
  Delay{1..9} (9 alike) : Delay  DelayLength=double(1)  InitialCondition=0  SampleTime=2.5e-07
  Relational Operator : RelationalOperator  Operator=<  OutDataTypeStr=boolean  SampleTime=2.5e-07  InputSameDT=off
  Switch : Switch  Criteria=u2 ~= 0  Threshold="fi(0,0,1,0,\"hex\",\"0\")"  OutDataTypeStr=fixdt(1, 25, 15)  SampleTime=2.5e-07  SaturateOnIntegerOverflow=off  InputSameDT=off
  Switch1 : Switch  Criteria=u2 ~= 0  Threshold="fi(0,0,1,0,\"hex\",\"0\")"  OutDataTypeStr=fixdt(0, 6, 0)  SampleTime=2.5e-07  SaturateOnIntegerOverflow=off  InputSameDT=off
  t : Demux  Outputs=2
  t1 : Demux  Outputs=2
  ValueOut : Outport  SampleTime=2.5e-07
  idxOut : Outport  Port=2  SampleTime=2.5e-07
  wires:
  Delay4/1 -> Switch/1
  Delay8/1 -> ValueOut/1
  valueIn/1 -> Delay3/1
  idxIn/1 -> Delay1/1
  Delay3/1 -> t1/1
  Delay1/1 -> t/1
  Switch1/1 -> Delay9/1
  t1/1 -> Delay4/1, Relational Operator/1
  Relational Operator/1 -> Delay2/1
  t1/2 -> Delay5/1, Relational Operator/2
  t/1 -> Delay6/1
  t/2 -> Delay7/1
  Delay5/1 -> Switch/3
  Delay2/1 -> Switch/2, Switch1/2
  Delay6/1 -> Switch1/1
  Delay7/1 -> Switch1/3
  Switch/1 -> Delay8/1
  Delay9/1 -> idxOut/1

== system gm_soc_dvbs2_fpga/DVBS2/DVBS2 TxRx/DVB-S2 HDL Receiver/Synchronizer and PL Header Decoder/PL Header Recovery/PL Header Decoder/ML Decoder/Get Min Index/For Each Subsystem_instance26 ==
  note: For Each
  valueIn : Inport  OutDataTypeStr=fixdt(1, 25, 15)  PortDimensions=[2]  SampleTime=2.5e-07
  idxIn : Inport  Port=2  OutDataTypeStr=fixdt(0, 6, 0)  PortDimensions=[2]  SampleTime=2.5e-07
  Delay{1..9} (9 alike) : Delay  DelayLength=double(1)  InitialCondition=0  SampleTime=2.5e-07
  Relational Operator : RelationalOperator  Operator=<  OutDataTypeStr=boolean  SampleTime=2.5e-07  InputSameDT=off
  Switch : Switch  Criteria=u2 ~= 0  Threshold="fi(0,0,1,0,\"hex\",\"0\")"  OutDataTypeStr=fixdt(1, 25, 15)  SampleTime=2.5e-07  SaturateOnIntegerOverflow=off  InputSameDT=off
  Switch1 : Switch  Criteria=u2 ~= 0  Threshold="fi(0,0,1,0,\"hex\",\"0\")"  OutDataTypeStr=fixdt(0, 6, 0)  SampleTime=2.5e-07  SaturateOnIntegerOverflow=off  InputSameDT=off
  t : Demux  Outputs=2
  t1 : Demux  Outputs=2
  ValueOut : Outport  SampleTime=2.5e-07
  idxOut : Outport  Port=2  SampleTime=2.5e-07
  wires:
  Delay8/1 -> ValueOut/1
  valueIn/1 -> Delay3/1
  Delay1/1 -> t/1
  Switch1/1 -> Delay9/1
  t1/1 -> Relational Operator/1, Delay4/1
  Delay3/1 -> t1/1
  idxIn/1 -> Delay1/1
  Relational Operator/1 -> Delay2/1
  t1/2 -> Delay5/1, Relational Operator/2
  Delay4/1 -> Switch/1
  t/1 -> Delay6/1
  t/2 -> Delay7/1
  Delay5/1 -> Switch/3
  Delay2/1 -> Switch/2, Switch1/2
  Delay6/1 -> Switch1/1
  Delay7/1 -> Switch1/3
  Switch/1 -> Delay8/1
  Delay9/1 -> idxOut/1

== system gm_soc_dvbs2_fpga/DVBS2/DVBS2 TxRx/DVB-S2 HDL Receiver/Synchronizer and PL Header Decoder/PL Header Recovery/PL Header Decoder/ML Decoder/Get Min Index/For Each Subsystem_instance27 ==
  note: For Each
  valueIn : Inport  OutDataTypeStr=fixdt(1, 25, 15)  PortDimensions=[2]  SampleTime=2.5e-07
  idxIn : Inport  Port=2  OutDataTypeStr=fixdt(0, 6, 0)  PortDimensions=[2]  SampleTime=2.5e-07
  Delay{1..9} (9 alike) : Delay  DelayLength=double(1)  InitialCondition=0  SampleTime=2.5e-07
  Relational Operator : RelationalOperator  Operator=<  OutDataTypeStr=boolean  SampleTime=2.5e-07  InputSameDT=off
  Switch : Switch  Criteria=u2 ~= 0  Threshold="fi(0,0,1,0,\"hex\",\"0\")"  OutDataTypeStr=fixdt(1, 25, 15)  SampleTime=2.5e-07  SaturateOnIntegerOverflow=off  InputSameDT=off
  Switch1 : Switch  Criteria=u2 ~= 0  Threshold="fi(0,0,1,0,\"hex\",\"0\")"  OutDataTypeStr=fixdt(0, 6, 0)  SampleTime=2.5e-07  SaturateOnIntegerOverflow=off  InputSameDT=off
  t : Demux  Outputs=2
  t1 : Demux  Outputs=2
  ValueOut : Outport  SampleTime=2.5e-07
  idxOut : Outport  Port=2  SampleTime=2.5e-07
  wires:
  valueIn/1 -> Delay3/1
  Delay1/1 -> t/1
  Delay3/1 -> t1/1
  idxIn/1 -> Delay1/1
  t1/1 -> Delay4/1, Relational Operator/1
  t1/2 -> Delay5/1, Relational Operator/2
  Relational Operator/1 -> Delay2/1
  Delay4/1 -> Switch/1
  t/1 -> Delay6/1
  t/2 -> Delay7/1
  Delay5/1 -> Switch/3
  Delay2/1 -> Switch/2, Switch1/2
  Delay6/1 -> Switch1/1
  Switch1/1 -> Delay9/1
  Delay7/1 -> Switch1/3
  Delay8/1 -> ValueOut/1
  Switch/1 -> Delay8/1
  Delay9/1 -> idxOut/1

== system gm_soc_dvbs2_fpga/DVBS2/DVBS2 TxRx/DVB-S2 HDL Receiver/Synchronizer and PL Header Decoder/PL Header Recovery/PL Header Decoder/ML Decoder/Get Min Index/For Each Subsystem_instance28 ==
  note: For Each
  valueIn : Inport  OutDataTypeStr=fixdt(1, 25, 15)  PortDimensions=[2]  SampleTime=2.5e-07
  idxIn : Inport  Port=2  OutDataTypeStr=fixdt(0, 6, 0)  PortDimensions=[2]  SampleTime=2.5e-07
  Delay{1..9} (9 alike) : Delay  DelayLength=double(1)  InitialCondition=0  SampleTime=2.5e-07
  Relational Operator : RelationalOperator  Operator=<  OutDataTypeStr=boolean  SampleTime=2.5e-07  InputSameDT=off
  Switch : Switch  Criteria=u2 ~= 0  Threshold="fi(0,0,1,0,\"hex\",\"0\")"  OutDataTypeStr=fixdt(1, 25, 15)  SampleTime=2.5e-07  SaturateOnIntegerOverflow=off  InputSameDT=off
  Switch1 : Switch  Criteria=u2 ~= 0  Threshold="fi(0,0,1,0,\"hex\",\"0\")"  OutDataTypeStr=fixdt(0, 6, 0)  SampleTime=2.5e-07  SaturateOnIntegerOverflow=off  InputSameDT=off
  t : Demux  Outputs=2
  t1 : Demux  Outputs=2
  ValueOut : Outport  SampleTime=2.5e-07
  idxOut : Outport  Port=2  SampleTime=2.5e-07
  wires:
  Delay4/1 -> Switch/1
  Delay8/1 -> ValueOut/1
  valueIn/1 -> Delay3/1
  Delay1/1 -> t/1
  Switch1/1 -> Delay9/1
  t1/1 -> Relational Operator/1, Delay4/1
  Delay3/1 -> t1/1
  idxIn/1 -> Delay1/1
  Relational Operator/1 -> Delay2/1
  t1/2 -> Delay5/1, Relational Operator/2
  t/1 -> Delay6/1
  t/2 -> Delay7/1
  Delay5/1 -> Switch/3
  Delay2/1 -> Switch/2, Switch1/2
  Delay6/1 -> Switch1/1
  Delay7/1 -> Switch1/3
  Switch/1 -> Delay8/1
  Delay9/1 -> idxOut/1
